simulink model "simlink"  (R2022b)
settings: Solver=VariableStepAuto  StartTime=0.0  StopTime=10.0  RelTol=1e-3
values from neighbouring files (symbols this model uses):
  x = [x, zeros(1,L-M)]    [task1.m]    (also in task2.m = [1,2,3,4]; task3.m = [x,zeros(1,L-M)]; task4.m = [1,1,1,1,1,1,1,1])
settings Model: Creator=ECAD -24  LastModifiedBy=ECAD -24

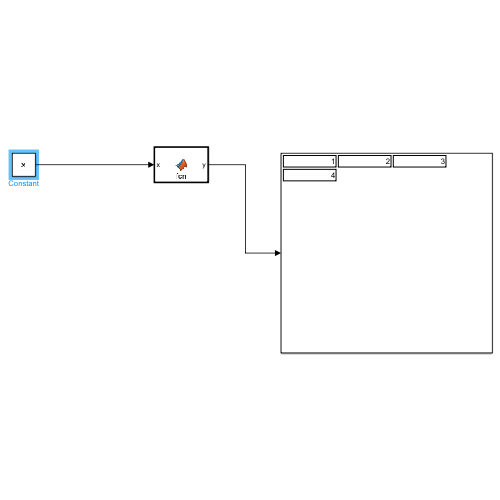
[thumbnail: Simulink's stored preview of the top-level diagram]
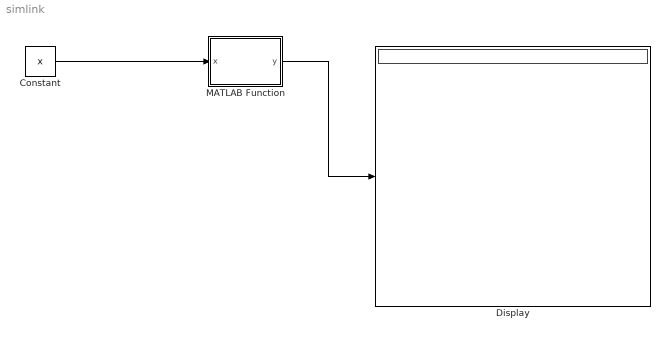
== system simlink ==
  Constant : Constant  Value=x
  Display : Display
  MATLAB Function : MATLAB Function  TreatAsAtomicUnit=on
  wires:
  Constant/1 -> MATLAB Function/1(x)
  MATLAB Function/1(y) -> Display/1

== matlab function simlink/MATLAB Function ==
  data: x input; y output
function y = fcn(x)

x = [1,2,3,4];
h = [2,1,2,1];

M = length(x);
N = length(h);
H = zeros(N,N);

x2 = [0,0,0,0,0,0,0,0,0,0];
h2 = [2,1,2,1,0,0,0,0,0,0];

for i=1:10
    x2(i) = 0.5.^(i-1);
end

M2 = length(x2);
N2 = length(h2);
H2 = zeros(N,N);


for n=1:N
    for i=1:N
        index = mod((n-i),N)+1;
        H(n,i) = h(index);
    end
end
Y = cconv(x,h,4);
Y2 = cconv(x2,h2,10);

y = x';
